simulink model "CRITIS_1_full"  (R2022b)
settings: Solver=VariableStepAuto  StartTime=0.0  StopTime=7  RelTol=1e-3
(part 10 of 13)

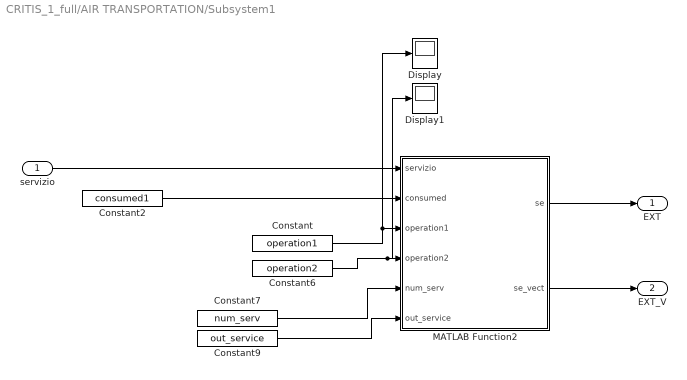
== system CRITIS_1_full/AIR TRANSPORTATION/Subsystem1 ==
  servizio : Inport
  Constant : Constant  Value=operation1
  Constant2 : Constant  Value=consumed1
  Constant6 : Constant  Value=operation2
  Constant7 : Constant  Value=num_serv
  Constant9 : Constant  Value=out_service
  Display : Display
  Display1 : Display
  MATLAB Function2 : MATLAB Function  TreatAsAtomicUnit=on
  EXT : Outport
  EXT_V : Outport  Port=2
  wires:
  Constant7/1 -> MATLAB Function2/5(num_serv)
  Constant9/1 -> MATLAB Function2/6(out_service)
  servizio/1 -> MATLAB Function2/1(servizio)
  Constant/1 -> Display/1, MATLAB Function2/3(operation1)
  Constant6/1 -> Display1/1, MATLAB Function2/4(operation2)
  MATLAB Function2/1(se) -> EXT/1
  MATLAB Function2/2(se_vect) -> EXT_V/1
  Constant2/1 -> MATLAB Function2/2(consumed)

== system CRITIS_1_full/AIR TRANSPORTATION/Subsystem10 ==
  servizio : Inport
  Constant : Constant  Value=operation1
  Constant2 : Constant  Value=consumed1
  Constant6 : Constant  Value=operation2
  Constant7 : Constant  Value=num_serv
  Constant9 : Constant  Value=out_service
  MATLAB Function2 : MATLAB Function  TreatAsAtomicUnit=on
  EXT : Outport
  EXT_V : Outport  Port=2
  wires:
  Constant7/1 -> MATLAB Function2/5(num_serv)
  Constant9/1 -> MATLAB Function2/6(out_service)
  servizio/1 -> MATLAB Function2/1(servizio)
  Constant/1 -> MATLAB Function2/3(operation1)
  Constant6/1 -> MATLAB Function2/4(operation2)
  MATLAB Function2/1(se) -> EXT/1
  MATLAB Function2/2(se_vect) -> EXT_V/1
  Constant2/1 -> MATLAB Function2/2(consumed)

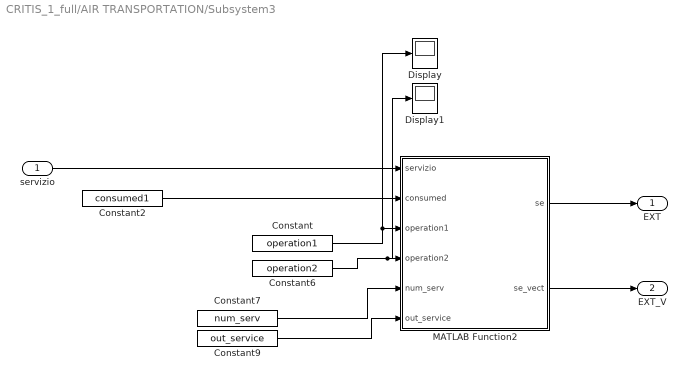
== system CRITIS_1_full/AIR TRANSPORTATION/Subsystem3 ==
  servizio : Inport
  Constant : Constant  Value=operation1
  Constant2 : Constant  Value=consumed1
  Constant6 : Constant  Value=operation2
  Constant7 : Constant  Value=num_serv
  Constant9 : Constant  Value=out_service
  Display : Display
  Display1 : Display
  MATLAB Function2 : MATLAB Function  TreatAsAtomicUnit=on
  EXT : Outport
  EXT_V : Outport  Port=2
  wires:
  Constant7/1 -> MATLAB Function2/5(num_serv)
  Constant9/1 -> MATLAB Function2/6(out_service)
  servizio/1 -> MATLAB Function2/1(servizio)
  Constant/1 -> Display/1, MATLAB Function2/3(operation1)
  Constant6/1 -> Display1/1, MATLAB Function2/4(operation2)
  MATLAB Function2/1(se) -> EXT/1
  MATLAB Function2/2(se_vect) -> EXT_V/1
  Constant2/1 -> MATLAB Function2/2(consumed)

== system CRITIS_1_full/AIR TRANSPORTATION/Subsystem4 ==
  servizio : Inport
  Constant : Constant  Value=operation1
  Constant2 : Constant  Value=consumed1
  Constant6 : Constant  Value=operation2
  Constant7 : Constant  Value=num_serv
  Constant9 : Constant  Value=out_service
  Display : Display
  Display1 : Display
  MATLAB Function2 : MATLAB Function  TreatAsAtomicUnit=on
  EXT : Outport
  EXT_V : Outport  Port=2
  wires:
  Constant7/1 -> MATLAB Function2/5(num_serv)
  Constant9/1 -> MATLAB Function2/6(out_service)
  servizio/1 -> MATLAB Function2/1(servizio)
  Constant/1 -> Display/1, MATLAB Function2/3(operation1)
  Constant6/1 -> Display1/1, MATLAB Function2/4(operation2)
  MATLAB Function2/1(se) -> EXT/1
  MATLAB Function2/2(se_vect) -> EXT_V/1
  Constant2/1 -> MATLAB Function2/2(consumed)

== system CRITIS_1_full/AIR TRANSPORTATION/Subsystem5 ==
  servizio : Inport
  Constant : Constant  Value=operation1
  Constant2 : Constant  Value=consumed1
  Constant6 : Constant  Value=operation2
  Constant7 : Constant  Value=num_serv
  Constant9 : Constant  Value=out_service
  Display : Display
  Display1 : Display
  MATLAB Function2 : MATLAB Function  TreatAsAtomicUnit=on
  EXT : Outport
  EXT_V : Outport  Port=2
  wires:
  Constant7/1 -> MATLAB Function2/5(num_serv)
  Constant9/1 -> MATLAB Function2/6(out_service)
  servizio/1 -> MATLAB Function2/1(servizio)
  Constant/1 -> Display/1, MATLAB Function2/3(operation1)
  Constant6/1 -> Display1/1, MATLAB Function2/4(operation2)
  MATLAB Function2/1(se) -> EXT/1
  MATLAB Function2/2(se_vect) -> EXT_V/1
  Constant2/1 -> MATLAB Function2/2(consumed)

== system CRITIS_1_full/AIR TRANSPORTATION/Subsystem6 ==
  servizio : Inport
  Constant : Constant  Value=operation1
  Constant2 : Constant  Value=consumed1
  Constant6 : Constant  Value=operation2
  Constant7 : Constant  Value=num_serv
  Constant9 : Constant  Value=out_service
  Display : Display
  Display1 : Display
  MATLAB Function2 : MATLAB Function  TreatAsAtomicUnit=on
  EXT : Outport
  EXT_V : Outport  Port=2
  wires:
  Constant7/1 -> MATLAB Function2/5(num_serv)
  Constant9/1 -> MATLAB Function2/6(out_service)
  servizio/1 -> MATLAB Function2/1(servizio)
  Constant/1 -> Display/1, MATLAB Function2/3(operation1)
  Constant6/1 -> Display1/1, MATLAB Function2/4(operation2)
  MATLAB Function2/1(se) -> EXT/1
  MATLAB Function2/2(se_vect) -> EXT_V/1
  Constant2/1 -> MATLAB Function2/2(consumed)

== system CRITIS_1_full/AIR TRANSPORTATION/Subsystem7 ==
  servizio : Inport
  Constant : Constant  Value=operation1
  Constant2 : Constant  Value=consumed1
  Constant6 : Constant  Value=operation2
  Constant7 : Constant  Value=num_serv
  Constant9 : Constant  Value=out_service
  Display : Display
  Display1 : Display
  MATLAB Function2 : MATLAB Function  TreatAsAtomicUnit=on
  EXT : Outport
  EXT_V : Outport  Port=2
  wires:
  Constant7/1 -> MATLAB Function2/5(num_serv)
  Constant9/1 -> MATLAB Function2/6(out_service)
  servizio/1 -> MATLAB Function2/1(servizio)
  Constant/1 -> Display/1, MATLAB Function2/3(operation1)
  Constant6/1 -> Display1/1, MATLAB Function2/4(operation2)
  MATLAB Function2/1(se) -> EXT/1
  MATLAB Function2/2(se_vect) -> EXT_V/1
  Constant2/1 -> MATLAB Function2/2(consumed)

== system CRITIS_1_full/AIR TRANSPORTATION/Subsystem8 ==
  servizio : Inport
  Constant : Constant  Value=operation1
  Constant2 : Constant  Value=consumed1
  Constant6 : Constant  Value=operation2
  Constant7 : Constant  Value=num_serv
  Constant9 : Constant  Value=out_service
  Display : Display
  Display1 : Display
  MATLAB Function2 : MATLAB Function  TreatAsAtomicUnit=on
  EXT : Outport
  EXT_V : Outport  Port=2
  wires:
  Constant7/1 -> MATLAB Function2/5(num_serv)
  Constant9/1 -> MATLAB Function2/6(out_service)
  servizio/1 -> MATLAB Function2/1(servizio)
  Constant/1 -> Display/1, MATLAB Function2/3(operation1)
  Constant6/1 -> Display1/1, MATLAB Function2/4(operation2)
  MATLAB Function2/1(se) -> EXT/1
  MATLAB Function2/2(se_vect) -> EXT_V/1
  Constant2/1 -> MATLAB Function2/2(consumed)

== system CRITIS_1_full/AIR TRANSPORTATION/Subsystem9 ==
  servizio : Inport
  Constant : Constant  Value=operation1
  Constant2 : Constant  Value=consumed1
  Constant6 : Constant  Value=operation2
  Constant7 : Constant  Value=num_serv
  Constant9 : Constant  Value=out_service
  MATLAB Function2 : MATLAB Function  TreatAsAtomicUnit=on
  EXT : Outport
  EXT_V : Outport  Port=2
  wires:
  Constant7/1 -> MATLAB Function2/5(num_serv)
  Constant9/1 -> MATLAB Function2/6(out_service)
  servizio/1 -> MATLAB Function2/1(servizio)
  Constant/1 -> MATLAB Function2/3(operation1)
  Constant6/1 -> MATLAB Function2/4(operation2)
  MATLAB Function2/1(se) -> EXT/1
  MATLAB Function2/2(se_vect) -> EXT_V/1
  Constant2/1 -> MATLAB Function2/2(consumed)

== system CRITIS_1_full/AIR TRANSPORTATION/delay ==
  in : Inport
  Clock : Clock
  Constant17 : Constant  Value=output
  Switch : Switch  Criteria=u2 > Threshold  Threshold=delay  SaturateOnIntegerOverflow=off  InputSameDT=off
  out : Outport
  wires:
  Switch/1 -> out/1
  Constant17/1 -> Switch/3
  in/1 -> Switch/1
  Clock/1 -> Switch/2

== system CRITIS_1_full/AIR TRANSPORTATION/delay1 ==
  in : Inport
  Clock : Clock
  Constant17 : Constant  Value=output
  Switch : Switch  Criteria=u2 > Threshold  Threshold=delay  SaturateOnIntegerOverflow=off  InputSameDT=off
  out : Outport
  wires:
  Switch/1 -> out/1
  Constant17/1 -> Switch/3
  in/1 -> Switch/1
  Clock/1 -> Switch/2

== system CRITIS_1_full/BANK 1/Subsystem1 ==
  servizio : Inport
  Constant : Constant  Value=operation1
  Constant2 : Constant  Value=consumed1
  Constant6 : Constant  Value=operation2
  Constant7 : Constant  Value=num_serv
  Constant9 : Constant  Value=out_service
  Display : Display
  Display1 : Display
  MATLAB Function2 : MATLAB Function  TreatAsAtomicUnit=on
  EXT : Outport
  EXT_V : Outport  Port=2
  wires:
  Constant7/1 -> MATLAB Function2/5(num_serv)
  Constant9/1 -> MATLAB Function2/6(out_service)
  servizio/1 -> MATLAB Function2/1(servizio)
  Constant/1 -> Display/1, MATLAB Function2/3(operation1)
  Constant6/1 -> Display1/1, MATLAB Function2/4(operation2)
  MATLAB Function2/1(se) -> EXT/1
  MATLAB Function2/2(se_vect) -> EXT_V/1
  Constant2/1 -> MATLAB Function2/2(consumed)

== system CRITIS_1_full/BANK 1/Subsystem2 ==
  servizio : Inport
  Constant : Constant  Value=operation1
  Constant2 : Constant  Value=consumed1
  Constant6 : Constant  Value=operation2
  Constant7 : Constant  Value=num_serv
  Constant9 : Constant  Value=out_service
  Display : Display
  Display1 : Display
  MATLAB Function2 : MATLAB Function  TreatAsAtomicUnit=on
  EXT : Outport
  EXT_V : Outport  Port=2
  wires:
  Constant7/1 -> MATLAB Function2/5(num_serv)
  Constant9/1 -> MATLAB Function2/6(out_service)
  servizio/1 -> MATLAB Function2/1(servizio)
  Constant/1 -> Display/1, MATLAB Function2/3(operation1)
  Constant6/1 -> Display1/1, MATLAB Function2/4(operation2)
  MATLAB Function2/1(se) -> EXT/1
  MATLAB Function2/2(se_vect) -> EXT_V/1
  Constant2/1 -> MATLAB Function2/2(consumed)

== system CRITIS_1_full/BANK 1/Subsystem3 ==
  servizio : Inport
  Constant : Constant  Value=operation1
  Constant2 : Constant  Value=consumed1
  Constant6 : Constant  Value=operation2
  Constant7 : Constant  Value=num_serv
  Constant9 : Constant  Value=out_service
  Display : Display
  Display1 : Display
  MATLAB Function2 : MATLAB Function  TreatAsAtomicUnit=on
  EXT : Outport
  EXT_V : Outport  Port=2
  wires:
  Constant7/1 -> MATLAB Function2/5(num_serv)
  Constant9/1 -> MATLAB Function2/6(out_service)
  servizio/1 -> MATLAB Function2/1(servizio)
  Constant/1 -> Display/1, MATLAB Function2/3(operation1)
  Constant6/1 -> Display1/1, MATLAB Function2/4(operation2)
  MATLAB Function2/1(se) -> EXT/1
  MATLAB Function2/2(se_vect) -> EXT_V/1
  Constant2/1 -> MATLAB Function2/2(consumed)

== system CRITIS_1_full/BANK 1/Subsystem4 ==
  servizio : Inport
  Constant : Constant  Value=operation1
  Constant2 : Constant  Value=consumed1
  Constant6 : Constant  Value=operation2
  Constant7 : Constant  Value=num_serv
  Constant9 : Constant  Value=out_service
  Display : Display
  Display1 : Display
  MATLAB Function2 : MATLAB Function  TreatAsAtomicUnit=on
  EXT : Outport
  EXT_V : Outport  Port=2
  wires:
  Constant7/1 -> MATLAB Function2/5(num_serv)
  Constant9/1 -> MATLAB Function2/6(out_service)
  servizio/1 -> MATLAB Function2/1(servizio)
  Constant/1 -> Display/1, MATLAB Function2/3(operation1)
  Constant6/1 -> Display1/1, MATLAB Function2/4(operation2)
  MATLAB Function2/1(se) -> EXT/1
  MATLAB Function2/2(se_vect) -> EXT_V/1
  Constant2/1 -> MATLAB Function2/2(consumed)

== system CRITIS_1_full/BANK 1/Subsystem5 ==
  servizio : Inport
  Constant : Constant  Value=operation1
  Constant2 : Constant  Value=consumed1
  Constant6 : Constant  Value=operation2
  Constant7 : Constant  Value=num_serv
  Constant9 : Constant  Value=out_service
  Display : Display
  Display1 : Display
  MATLAB Function2 : MATLAB Function  TreatAsAtomicUnit=on
  EXT : Outport
  EXT_V : Outport  Port=2
  wires:
  Constant7/1 -> MATLAB Function2/5(num_serv)
  Constant9/1 -> MATLAB Function2/6(out_service)
  servizio/1 -> MATLAB Function2/1(servizio)
  Constant/1 -> Display/1, MATLAB Function2/3(operation1)
  Constant6/1 -> Display1/1, MATLAB Function2/4(operation2)
  MATLAB Function2/1(se) -> EXT/1
  MATLAB Function2/2(se_vect) -> EXT_V/1
  Constant2/1 -> MATLAB Function2/2(consumed)

== system CRITIS_1_full/BANK 1/Subsystem6 ==
  servizio : Inport
  Constant : Constant  Value=operation1
  Constant2 : Constant  Value=consumed1
  Constant6 : Constant  Value=operation2
  Constant7 : Constant  Value=num_serv
  Constant9 : Constant  Value=out_service
  Display : Display
  Display1 : Display
  MATLAB Function2 : MATLAB Function  TreatAsAtomicUnit=on
  EXT : Outport
  EXT_V : Outport  Port=2
  wires:
  Constant7/1 -> MATLAB Function2/5(num_serv)
  Constant9/1 -> MATLAB Function2/6(out_service)
  servizio/1 -> MATLAB Function2/1(servizio)
  Constant/1 -> Display/1, MATLAB Function2/3(operation1)
  Constant6/1 -> Display1/1, MATLAB Function2/4(operation2)
  MATLAB Function2/1(se) -> EXT/1
  MATLAB Function2/2(se_vect) -> EXT_V/1
  Constant2/1 -> MATLAB Function2/2(consumed)

== system CRITIS_1_full/BANK 1/delay ==
  in : Inport
  Clock : Clock
  Constant17 : Constant  Value=output
  Switch : Switch  Criteria=u2 > Threshold  Threshold=delay  SaturateOnIntegerOverflow=off  InputSameDT=off
  out : Outport
  wires:
  Switch/1 -> out/1
  Constant17/1 -> Switch/3
  in/1 -> Switch/1
  Clock/1 -> Switch/2

== system CRITIS_1_full/BANK 1/delay1 ==
  in : Inport
  Clock : Clock
  Constant17 : Constant  Value=output
  Switch : Switch  Criteria=u2 > Threshold  Threshold=delay  SaturateOnIntegerOverflow=off  InputSameDT=off
  out : Outport
  wires:
  Switch/1 -> out/1
  Constant17/1 -> Switch/3
  in/1 -> Switch/1
  Clock/1 -> Switch/2

== system CRITIS_1_full/DEPARTMENT OF INDUSTRIAL DEVELOPMENT/Subsystem1 ==
  servizio : Inport
  Constant : Constant  Value=operation1
  Constant2 : Constant  Value=consumed1
  Constant6 : Constant  Value=operation2
  Constant7 : Constant  Value=num_serv
  Constant9 : Constant  Value=out_service
  Display : Display
  Display1 : Display
  MATLAB Function2 : MATLAB Function  TreatAsAtomicUnit=on
  EXT : Outport
  EXT_V : Outport  Port=2
  wires:
  Constant7/1 -> MATLAB Function2/5(num_serv)
  Constant9/1 -> MATLAB Function2/6(out_service)
  servizio/1 -> MATLAB Function2/1(servizio)
  Constant/1 -> Display/1, MATLAB Function2/3(operation1)
  Constant6/1 -> Display1/1, MATLAB Function2/4(operation2)
  MATLAB Function2/1(se) -> EXT/1
  MATLAB Function2/2(se_vect) -> EXT_V/1
  Constant2/1 -> MATLAB Function2/2(consumed)

== system CRITIS_1_full/DEPARTMENT OF INDUSTRIAL DEVELOPMENT/Subsystem2 ==
  servizio : Inport
  Constant : Constant  Value=operation1
  Constant2 : Constant  Value=consumed1
  Constant6 : Constant  Value=operation2
  Constant7 : Constant  Value=num_serv
  Constant9 : Constant  Value=out_service
  Display : Display
  Display1 : Display
  MATLAB Function2 : MATLAB Function  TreatAsAtomicUnit=on
  EXT : Outport
  EXT_V : Outport  Port=2
  wires:
  Constant7/1 -> MATLAB Function2/5(num_serv)
  Constant9/1 -> MATLAB Function2/6(out_service)
  servizio/1 -> MATLAB Function2/1(servizio)
  Constant/1 -> Display/1, MATLAB Function2/3(operation1)
  Constant6/1 -> Display1/1, MATLAB Function2/4(operation2)
  MATLAB Function2/1(se) -> EXT/1
  MATLAB Function2/2(se_vect) -> EXT_V/1
  Constant2/1 -> MATLAB Function2/2(consumed)

== system CRITIS_1_full/DEPARTMENT OF INDUSTRIAL DEVELOPMENT/Subsystem3 ==
  servizio : Inport
  Constant : Constant  Value=operation1
  Constant2 : Constant  Value=consumed1
  Constant6 : Constant  Value=operation2
  Constant7 : Constant  Value=num_serv
  Constant9 : Constant  Value=out_service
  Display : Display
  Display1 : Display
  MATLAB Function2 : MATLAB Function  TreatAsAtomicUnit=on
  EXT : Outport
  EXT_V : Outport  Port=2
  wires:
  Constant7/1 -> MATLAB Function2/5(num_serv)
  Constant9/1 -> MATLAB Function2/6(out_service)
  servizio/1 -> MATLAB Function2/1(servizio)
  Constant/1 -> Display/1, MATLAB Function2/3(operation1)
  Constant6/1 -> Display1/1, MATLAB Function2/4(operation2)
  MATLAB Function2/1(se) -> EXT/1
  MATLAB Function2/2(se_vect) -> EXT_V/1
  Constant2/1 -> MATLAB Function2/2(consumed)

== system CRITIS_1_full/DEPARTMENT OF INDUSTRIAL DEVELOPMENT/Subsystem4 ==
  servizio : Inport
  Constant : Constant  Value=operation1
  Constant2 : Constant  Value=consumed1
  Constant6 : Constant  Value=operation2
  Constant7 : Constant  Value=num_serv
  Constant9 : Constant  Value=out_service
  Display : Display
  Display1 : Display
  MATLAB Function2 : MATLAB Function  TreatAsAtomicUnit=on
  EXT : Outport
  EXT_V : Outport  Port=2
  wires:
  Constant7/1 -> MATLAB Function2/5(num_serv)
  Constant9/1 -> MATLAB Function2/6(out_service)
  servizio/1 -> MATLAB Function2/1(servizio)
  Constant/1 -> Display/1, MATLAB Function2/3(operation1)
  Constant6/1 -> Display1/1, MATLAB Function2/4(operation2)
  MATLAB Function2/1(se) -> EXT/1
  MATLAB Function2/2(se_vect) -> EXT_V/1
  Constant2/1 -> MATLAB Function2/2(consumed)

== system CRITIS_1_full/DEPARTMENT OF INDUSTRIAL DEVELOPMENT/Subsystem5 ==
  servizio : Inport
  Constant : Constant  Value=operation1
  Constant2 : Constant  Value=consumed1
  Constant6 : Constant  Value=operation2
  Constant7 : Constant  Value=num_serv
  Constant9 : Constant  Value=out_service
  Display : Display
  Display1 : Display
  MATLAB Function2 : MATLAB Function  TreatAsAtomicUnit=on
  EXT : Outport
  EXT_V : Outport  Port=2
  wires:
  Constant7/1 -> MATLAB Function2/5(num_serv)
  Constant9/1 -> MATLAB Function2/6(out_service)
  servizio/1 -> MATLAB Function2/1(servizio)
  Constant/1 -> Display/1, MATLAB Function2/3(operation1)
  Constant6/1 -> Display1/1, MATLAB Function2/4(operation2)
  MATLAB Function2/1(se) -> EXT/1
  MATLAB Function2/2(se_vect) -> EXT_V/1
  Constant2/1 -> MATLAB Function2/2(consumed)

== system CRITIS_1_full/DEPARTMENT OF INDUSTRIAL DEVELOPMENT/Subsystem6 ==
  servizio : Inport
  Constant : Constant  Value=operation1
  Constant2 : Constant  Value=consumed1
  Constant6 : Constant  Value=operation2
  Constant7 : Constant  Value=num_serv
  Constant9 : Constant  Value=out_service
  Display : Display
  Display1 : Display
  MATLAB Function2 : MATLAB Function  TreatAsAtomicUnit=on
  EXT : Outport
  EXT_V : Outport  Port=2
  wires:
  Constant7/1 -> MATLAB Function2/5(num_serv)
  Constant9/1 -> MATLAB Function2/6(out_service)
  servizio/1 -> MATLAB Function2/1(servizio)
  Constant/1 -> Display/1, MATLAB Function2/3(operation1)
  Constant6/1 -> Display1/1, MATLAB Function2/4(operation2)
  MATLAB Function2/1(se) -> EXT/1
  MATLAB Function2/2(se_vect) -> EXT_V/1
  Constant2/1 -> MATLAB Function2/2(consumed)

== system CRITIS_1_full/DEPARTMENT OF INDUSTRIAL DEVELOPMENT/delay ==
  in : Inport
  Clock : Clock
  Constant17 : Constant  Value=output
  Switch : Switch  Criteria=u2 > Threshold  Threshold=delay  SaturateOnIntegerOverflow=off  InputSameDT=off
  out : Outport
  wires:
  Switch/1 -> out/1
  Constant17/1 -> Switch/3
  in/1 -> Switch/1
  Clock/1 -> Switch/2

== system CRITIS_1_full/DEPARTMENT OF INDUSTRIAL DEVELOPMENT/delay1 ==
  in : Inport
  Clock : Clock
  Constant17 : Constant  Value=output
  Switch : Switch  Criteria=u2 > Threshold  Threshold=delay  SaturateOnIntegerOverflow=off  InputSameDT=off
  out : Outport
  wires:
  Switch/1 -> out/1
  Constant17/1 -> Switch/3
  in/1 -> Switch/1
  Clock/1 -> Switch/2

== system CRITIS_1_full/ENERGY PROVIDER 1/Subsystem1 ==
  servizio : Inport
  Constant : Constant  Value=operation1
  Constant2 : Constant  Value=consumed1
  Constant6 : Constant  Value=operation2
  Constant7 : Constant  Value=num_serv
  Constant9 : Constant  Value=out_service
  MATLAB Function2 : MATLAB Function  TreatAsAtomicUnit=on
  EXT : Outport
  EXT_V : Outport  Port=2
  wires:
  Constant7/1 -> MATLAB Function2/5(num_serv)
  Constant9/1 -> MATLAB Function2/6(out_service)
  servizio/1 -> MATLAB Function2/1(servizio)
  Constant/1 -> MATLAB Function2/3(operation1)
  Constant6/1 -> MATLAB Function2/4(operation2)
  MATLAB Function2/1(se) -> EXT/1
  MATLAB Function2/2(se_vect) -> EXT_V/1
  Constant2/1 -> MATLAB Function2/2(consumed)

== system CRITIS_1_full/ENERGY PROVIDER 1/Subsystem10 ==
  servizio : Inport
  Constant : Constant  Value=operation1
  Constant2 : Constant  Value=consumed1
  Constant6 : Constant  Value=operation2
  Constant7 : Constant  Value=num_serv
  Constant9 : Constant  Value=out_service
  MATLAB Function2 : MATLAB Function  TreatAsAtomicUnit=on
  EXT : Outport
  EXT_V : Outport  Port=2
  wires:
  Constant7/1 -> MATLAB Function2/5(num_serv)
  Constant9/1 -> MATLAB Function2/6(out_service)
  servizio/1 -> MATLAB Function2/1(servizio)
  Constant/1 -> MATLAB Function2/3(operation1)
  Constant6/1 -> MATLAB Function2/4(operation2)
  MATLAB Function2/1(se) -> EXT/1
  MATLAB Function2/2(se_vect) -> EXT_V/1
  Constant2/1 -> MATLAB Function2/2(consumed)

== system CRITIS_1_full/ENERGY PROVIDER 1/Subsystem2 ==
  servizio : Inport
  Constant : Constant  Value=operation1
  Constant2 : Constant  Value=consumed1
  Constant6 : Constant  Value=operation2
  Constant7 : Constant  Value=num_serv
  Constant9 : Constant  Value=out_service
  MATLAB Function2 : MATLAB Function  TreatAsAtomicUnit=on
  EXT : Outport
  EXT_V : Outport  Port=2
  wires:
  Constant7/1 -> MATLAB Function2/5(num_serv)
  Constant9/1 -> MATLAB Function2/6(out_service)
  servizio/1 -> MATLAB Function2/1(servizio)
  Constant/1 -> MATLAB Function2/3(operation1)
  Constant6/1 -> MATLAB Function2/4(operation2)
  MATLAB Function2/1(se) -> EXT/1
  MATLAB Function2/2(se_vect) -> EXT_V/1
  Constant2/1 -> MATLAB Function2/2(consumed)

== system CRITIS_1_full/ENERGY PROVIDER 1/Subsystem3 ==
  servizio : Inport
  Constant : Constant  Value=operation1
  Constant2 : Constant  Value=consumed1
  Constant6 : Constant  Value=operation2
  Constant7 : Constant  Value=num_serv
  Constant9 : Constant  Value=out_service
  Display : Display
  Display1 : Display
  MATLAB Function2 : MATLAB Function  TreatAsAtomicUnit=on
  EXT : Outport
  EXT_V : Outport  Port=2
  wires:
  Constant7/1 -> MATLAB Function2/5(num_serv)
  Constant9/1 -> MATLAB Function2/6(out_service)
  servizio/1 -> MATLAB Function2/1(servizio)
  Constant/1 -> Display/1, MATLAB Function2/3(operation1)
  Constant6/1 -> Display1/1, MATLAB Function2/4(operation2)
  MATLAB Function2/1(se) -> EXT/1
  MATLAB Function2/2(se_vect) -> EXT_V/1
  Constant2/1 -> MATLAB Function2/2(consumed)

== system CRITIS_1_full/ENERGY PROVIDER 1/Subsystem4 ==
  servizio : Inport
  Constant : Constant  Value=operation1
  Constant2 : Constant  Value=consumed1
  Constant6 : Constant  Value=operation2
  Constant7 : Constant  Value=num_serv
  Constant9 : Constant  Value=out_service
  MATLAB Function2 : MATLAB Function  TreatAsAtomicUnit=on
  EXT : Outport
  EXT_V : Outport  Port=2
  wires:
  Constant7/1 -> MATLAB Function2/5(num_serv)
  Constant9/1 -> MATLAB Function2/6(out_service)
  servizio/1 -> MATLAB Function2/1(servizio)
  Constant/1 -> MATLAB Function2/3(operation1)
  Constant6/1 -> MATLAB Function2/4(operation2)
  MATLAB Function2/1(se) -> EXT/1
  MATLAB Function2/2(se_vect) -> EXT_V/1
  Constant2/1 -> MATLAB Function2/2(consumed)

== system CRITIS_1_full/ENERGY PROVIDER 1/delay ==
  in : Inport
  Clock : Clock
  Constant17 : Constant  Value=output
  Switch : Switch  Criteria=u2 > Threshold  Threshold=delay  SaturateOnIntegerOverflow=off  InputSameDT=off
  out : Outport
  wires:
  Switch/1 -> out/1
  Constant17/1 -> Switch/3
  in/1 -> Switch/1
  Clock/1 -> Switch/2

== system CRITIS_1_full/ENERGY PROVIDER 1/delay1 ==
  in : Inport
  Clock : Clock
  Constant17 : Constant  Value=output
  Switch : Switch  Criteria=u2 > Threshold  Threshold=delay  SaturateOnIntegerOverflow=off  InputSameDT=off
  out : Outport
  wires:
  Switch/1 -> out/1
  Constant17/1 -> Switch/3
  in/1 -> Switch/1
  Clock/1 -> Switch/2

== system CRITIS_1_full/ENERGY PROVIDER 2/Subsystem1 ==
  servizio : Inport
  Constant : Constant  Value=operation1
  Constant2 : Constant  Value=consumed1
  Constant6 : Constant  Value=operation2
  Constant7 : Constant  Value=num_serv
  Constant9 : Constant  Value=out_service
  MATLAB Function2 : MATLAB Function  TreatAsAtomicUnit=on
  EXT : Outport
  EXT_V : Outport  Port=2
  wires:
  Constant7/1 -> MATLAB Function2/5(num_serv)
  Constant9/1 -> MATLAB Function2/6(out_service)
  servizio/1 -> MATLAB Function2/1(servizio)
  Constant/1 -> MATLAB Function2/3(operation1)
  Constant6/1 -> MATLAB Function2/4(operation2)
  MATLAB Function2/1(se) -> EXT/1
  MATLAB Function2/2(se_vect) -> EXT_V/1
  Constant2/1 -> MATLAB Function2/2(consumed)

== system CRITIS_1_full/ENERGY PROVIDER 2/Subsystem2 ==
  servizio : Inport
  Constant : Constant  Value=operation1
  Constant2 : Constant  Value=consumed1
  Constant6 : Constant  Value=operation2
  Constant7 : Constant  Value=num_serv
  Constant9 : Constant  Value=out_service
  MATLAB Function2 : MATLAB Function  TreatAsAtomicUnit=on
  EXT : Outport
  EXT_V : Outport  Port=2
  wires:
  Constant7/1 -> MATLAB Function2/5(num_serv)
  Constant9/1 -> MATLAB Function2/6(out_service)
  servizio/1 -> MATLAB Function2/1(servizio)
  Constant/1 -> MATLAB Function2/3(operation1)
  Constant6/1 -> MATLAB Function2/4(operation2)
  MATLAB Function2/1(se) -> EXT/1
  MATLAB Function2/2(se_vect) -> EXT_V/1
  Constant2/1 -> MATLAB Function2/2(consumed)

== system CRITIS_1_full/ENERGY PROVIDER 2/Subsystem4 ==
  servizio : Inport
  Constant : Constant  Value=operation1
  Constant2 : Constant  Value=consumed1
  Constant6 : Constant  Value=operation2
  Constant7 : Constant  Value=num_serv
  Constant9 : Constant  Value=out_service
  MATLAB Function2 : MATLAB Function  TreatAsAtomicUnit=on
  EXT : Outport
  EXT_V : Outport  Port=2
  wires:
  Constant7/1 -> MATLAB Function2/5(num_serv)
  Constant9/1 -> MATLAB Function2/6(out_service)
  servizio/1 -> MATLAB Function2/1(servizio)
  Constant/1 -> MATLAB Function2/3(operation1)
  Constant6/1 -> MATLAB Function2/4(operation2)
  MATLAB Function2/1(se) -> EXT/1
  MATLAB Function2/2(se_vect) -> EXT_V/1
  Constant2/1 -> MATLAB Function2/2(consumed)

== system CRITIS_1_full/ENERGY PROVIDER 2/Subsystem9 ==
  servizio : Inport
  Constant : Constant  Value=operation1
  Constant2 : Constant  Value=consumed1
  Constant6 : Constant  Value=operation2
  Constant7 : Constant  Value=num_serv
  Constant9 : Constant  Value=out_service
  MATLAB Function2 : MATLAB Function  TreatAsAtomicUnit=on
  EXT : Outport
  EXT_V : Outport  Port=2
  wires:
  Constant7/1 -> MATLAB Function2/5(num_serv)
  Constant9/1 -> MATLAB Function2/6(out_service)
  servizio/1 -> MATLAB Function2/1(servizio)
  Constant/1 -> MATLAB Function2/3(operation1)
  Constant6/1 -> MATLAB Function2/4(operation2)
  MATLAB Function2/1(se) -> EXT/1
  MATLAB Function2/2(se_vect) -> EXT_V/1
  Constant2/1 -> MATLAB Function2/2(consumed)

== system CRITIS_1_full/ENERGY PROVIDER 2/delay ==
  in : Inport
  Clock : Clock
  Constant17 : Constant  Value=output
  Switch : Switch  Criteria=u2 > Threshold  Threshold=delay  SaturateOnIntegerOverflow=off  InputSameDT=off
  out : Outport
  wires:
  Switch/1 -> out/1
  Constant17/1 -> Switch/3
  in/1 -> Switch/1
  Clock/1 -> Switch/2

== system CRITIS_1_full/ENERGY PROVIDER 2/delay1 ==
  in : Inport
  Clock : Clock
  Constant17 : Constant  Value=output
  Switch : Switch  Criteria=u2 > Threshold  Threshold=delay  SaturateOnIntegerOverflow=off  InputSameDT=off
  out : Outport
  wires:
  Switch/1 -> out/1
  Constant17/1 -> Switch/3
  in/1 -> Switch/1
  Clock/1 -> Switch/2

== system CRITIS_1_full/RAILWAYS/Subsystem1 ==
  servizio : Inport
  Constant : Constant  Value=operation1
  Constant2 : Constant  Value=consumed1
  Constant6 : Constant  Value=operation2
  Constant7 : Constant  Value=num_serv
  Constant9 : Constant  Value=out_service
  Display : Display
  Display1 : Display
  MATLAB Function2 : MATLAB Function  TreatAsAtomicUnit=on
  EXT : Outport
  EXT_V : Outport  Port=2
  wires:
  Constant7/1 -> MATLAB Function2/5(num_serv)
  Constant9/1 -> MATLAB Function2/6(out_service)
  servizio/1 -> MATLAB Function2/1(servizio)
  Constant/1 -> Display/1, MATLAB Function2/3(operation1)
  Constant6/1 -> Display1/1, MATLAB Function2/4(operation2)
  MATLAB Function2/1(se) -> EXT/1
  MATLAB Function2/2(se_vect) -> EXT_V/1
  Constant2/1 -> MATLAB Function2/2(consumed)

== system CRITIS_1_full/RAILWAYS/Subsystem10 ==
  servizio : Inport
  Constant : Constant  Value=operation1
  Constant2 : Constant  Value=consumed1
  Constant6 : Constant  Value=operation2
  Constant7 : Constant  Value=num_serv
  Constant9 : Constant  Value=out_service
  Display : Display
  Display1 : Display
  MATLAB Function2 : MATLAB Function  TreatAsAtomicUnit=on
  EXT : Outport
  EXT_V : Outport  Port=2
  wires:
  Constant7/1 -> MATLAB Function2/5(num_serv)
  Constant9/1 -> MATLAB Function2/6(out_service)
  servizio/1 -> MATLAB Function2/1(servizio)
  Constant/1 -> Display/1, MATLAB Function2/3(operation1)
  Constant6/1 -> Display1/1, MATLAB Function2/4(operation2)
  MATLAB Function2/1(se) -> EXT/1
  MATLAB Function2/2(se_vect) -> EXT_V/1
  Constant2/1 -> MATLAB Function2/2(consumed)

== system CRITIS_1_full/RAILWAYS/Subsystem11 ==
  servizio : Inport
  Constant : Constant  Value=operation1
  Constant2 : Constant  Value=consumed1
  Constant6 : Constant  Value=operation2
  Constant7 : Constant  Value=num_serv
  Constant9 : Constant  Value=out_service
  MATLAB Function2 : MATLAB Function  TreatAsAtomicUnit=on
  EXT : Outport
  EXT_V : Outport  Port=2
  wires:
  Constant7/1 -> MATLAB Function2/5(num_serv)
  Constant9/1 -> MATLAB Function2/6(out_service)
  servizio/1 -> MATLAB Function2/1(servizio)
  Constant/1 -> MATLAB Function2/3(operation1)
  Constant6/1 -> MATLAB Function2/4(operation2)
  MATLAB Function2/1(se) -> EXT/1
  MATLAB Function2/2(se_vect) -> EXT_V/1
  Constant2/1 -> MATLAB Function2/2(consumed)

== system CRITIS_1_full/RAILWAYS/Subsystem2 ==
  servizio : Inport
  Constant : Constant  Value=operation1
  Constant2 : Constant  Value=consumed1
  Constant6 : Constant  Value=operation2
  Constant7 : Constant  Value=num_serv
  Constant9 : Constant  Value=out_service
  Display : Display
  Display1 : Display
  MATLAB Function2 : MATLAB Function  TreatAsAtomicUnit=on
  EXT : Outport
  EXT_V : Outport  Port=2
  wires:
  Constant7/1 -> MATLAB Function2/5(num_serv)
  Constant9/1 -> MATLAB Function2/6(out_service)
  servizio/1 -> MATLAB Function2/1(servizio)
  Constant/1 -> Display/1, MATLAB Function2/3(operation1)
  Constant6/1 -> Display1/1, MATLAB Function2/4(operation2)
  MATLAB Function2/1(se) -> EXT/1
  MATLAB Function2/2(se_vect) -> EXT_V/1
  Constant2/1 -> MATLAB Function2/2(consumed)

== system CRITIS_1_full/RAILWAYS/Subsystem3 ==
  servizio : Inport
  Constant : Constant  Value=operation1
  Constant2 : Constant  Value=consumed1
  Constant6 : Constant  Value=operation2
  Constant7 : Constant  Value=num_serv
  Constant9 : Constant  Value=out_service
  Display : Display
  Display1 : Display
  MATLAB Function2 : MATLAB Function  TreatAsAtomicUnit=on
  EXT : Outport
  EXT_V : Outport  Port=2
  wires:
  Constant7/1 -> MATLAB Function2/5(num_serv)
  Constant9/1 -> MATLAB Function2/6(out_service)
  servizio/1 -> MATLAB Function2/1(servizio)
  Constant/1 -> Display/1, MATLAB Function2/3(operation1)
  Constant6/1 -> Display1/1, MATLAB Function2/4(operation2)
  MATLAB Function2/1(se) -> EXT/1
  MATLAB Function2/2(se_vect) -> EXT_V/1
  Constant2/1 -> MATLAB Function2/2(consumed)

== system CRITIS_1_full/RAILWAYS/Subsystem4 ==
  servizio : Inport
  Constant : Constant  Value=operation1
  Constant2 : Constant  Value=consumed1
  Constant6 : Constant  Value=operation2
  Constant7 : Constant  Value=num_serv
  Constant9 : Constant  Value=out_service
  Display : Display
  Display1 : Display
  MATLAB Function2 : MATLAB Function  TreatAsAtomicUnit=on
  EXT : Outport
  EXT_V : Outport  Port=2
  wires:
  Constant7/1 -> MATLAB Function2/5(num_serv)
  Constant9/1 -> MATLAB Function2/6(out_service)
  servizio/1 -> MATLAB Function2/1(servizio)
  Constant/1 -> Display/1, MATLAB Function2/3(operation1)
  Constant6/1 -> Display1/1, MATLAB Function2/4(operation2)
  MATLAB Function2/1(se) -> EXT/1
  MATLAB Function2/2(se_vect) -> EXT_V/1
  Constant2/1 -> MATLAB Function2/2(consumed)

== system CRITIS_1_full/RAILWAYS/Subsystem5 ==
  servizio : Inport
  Constant : Constant  Value=operation1
  Constant2 : Constant  Value=consumed1
  Constant6 : Constant  Value=operation2
  Constant7 : Constant  Value=num_serv
  Constant9 : Constant  Value=out_service
  Display : Display
  Display1 : Display
  MATLAB Function2 : MATLAB Function  TreatAsAtomicUnit=on
  EXT : Outport
  EXT_V : Outport  Port=2
  wires:
  Constant7/1 -> MATLAB Function2/5(num_serv)
  Constant9/1 -> MATLAB Function2/6(out_service)
  servizio/1 -> MATLAB Function2/1(servizio)
  Constant/1 -> Display/1, MATLAB Function2/3(operation1)
  Constant6/1 -> Display1/1, MATLAB Function2/4(operation2)
  MATLAB Function2/1(se) -> EXT/1
  MATLAB Function2/2(se_vect) -> EXT_V/1
  Constant2/1 -> MATLAB Function2/2(consumed)

== system CRITIS_1_full/RAILWAYS/Subsystem6 ==
  servizio : Inport
  Constant : Constant  Value=operation1
  Constant2 : Constant  Value=consumed1
  Constant6 : Constant  Value=operation2
  Constant7 : Constant  Value=num_serv
  Constant9 : Constant  Value=out_service
  Display : Display
  Display1 : Display
  MATLAB Function2 : MATLAB Function  TreatAsAtomicUnit=on
  EXT : Outport
  EXT_V : Outport  Port=2
  wires:
  Constant7/1 -> MATLAB Function2/5(num_serv)
  Constant9/1 -> MATLAB Function2/6(out_service)
  servizio/1 -> MATLAB Function2/1(servizio)
  Constant/1 -> Display/1, MATLAB Function2/3(operation1)
  Constant6/1 -> Display1/1, MATLAB Function2/4(operation2)
  MATLAB Function2/1(se) -> EXT/1
  MATLAB Function2/2(se_vect) -> EXT_V/1
  Constant2/1 -> MATLAB Function2/2(consumed)

== system CRITIS_1_full/RAILWAYS/Subsystem7 ==
  servizio : Inport
  Constant : Constant  Value=operation1
  Constant2 : Constant  Value=consumed1
  Constant6 : Constant  Value=operation2
  Constant7 : Constant  Value=num_serv
  Constant9 : Constant  Value=out_service
  Display : Display
  Display1 : Display
  MATLAB Function2 : MATLAB Function  TreatAsAtomicUnit=on
  EXT : Outport
  EXT_V : Outport  Port=2
  wires:
  Constant7/1 -> MATLAB Function2/5(num_serv)
  Constant9/1 -> MATLAB Function2/6(out_service)
  servizio/1 -> MATLAB Function2/1(servizio)
  Constant/1 -> Display/1, MATLAB Function2/3(operation1)
  Constant6/1 -> Display1/1, MATLAB Function2/4(operation2)
  MATLAB Function2/1(se) -> EXT/1
  MATLAB Function2/2(se_vect) -> EXT_V/1
  Constant2/1 -> MATLAB Function2/2(consumed)

== system CRITIS_1_full/RAILWAYS/Subsystem8 ==
  servizio : Inport
  Constant : Constant  Value=operation1
  Constant2 : Constant  Value=consumed1
  Constant6 : Constant  Value=operation2
  Constant7 : Constant  Value=num_serv
  Constant9 : Constant  Value=out_service
  Display : Display
  Display1 : Display
  MATLAB Function2 : MATLAB Function  TreatAsAtomicUnit=on
  EXT : Outport
  EXT_V : Outport  Port=2
  wires:
  Constant7/1 -> MATLAB Function2/5(num_serv)
  Constant9/1 -> MATLAB Function2/6(out_service)
  servizio/1 -> MATLAB Function2/1(servizio)
  Constant/1 -> Display/1, MATLAB Function2/3(operation1)
  Constant6/1 -> Display1/1, MATLAB Function2/4(operation2)
  MATLAB Function2/1(se) -> EXT/1
  MATLAB Function2/2(se_vect) -> EXT_V/1
  Constant2/1 -> MATLAB Function2/2(consumed)

== system CRITIS_1_full/RAILWAYS/Subsystem9 ==
  servizio : Inport
  Constant : Constant  Value=operation1
  Constant2 : Constant  Value=consumed1
  Constant6 : Constant  Value=operation2
  Constant7 : Constant  Value=num_serv
  Constant9 : Constant  Value=out_service
  Display : Display
  Display1 : Display
  MATLAB Function2 : MATLAB Function  TreatAsAtomicUnit=on
  EXT : Outport
  EXT_V : Outport  Port=2
  wires:
  Constant7/1 -> MATLAB Function2/5(num_serv)
  Constant9/1 -> MATLAB Function2/6(out_service)
  servizio/1 -> MATLAB Function2/1(servizio)
  Constant/1 -> Display/1, MATLAB Function2/3(operation1)
  Constant6/1 -> Display1/1, MATLAB Function2/4(operation2)
  MATLAB Function2/1(se) -> EXT/1
  MATLAB Function2/2(se_vect) -> EXT_V/1
  Constant2/1 -> MATLAB Function2/2(consumed)

== system CRITIS_1_full/RAILWAYS/delay ==
  in : Inport
  Clock : Clock
  Constant17 : Constant  Value=output
  Switch : Switch  Criteria=u2 > Threshold  Threshold=delay  SaturateOnIntegerOverflow=off  InputSameDT=off
  out : Outport
  wires:
  Switch/1 -> out/1
  Constant17/1 -> Switch/3
  in/1 -> Switch/1
  Clock/1 -> Switch/2

== system CRITIS_1_full/RAILWAYS/delay1 ==
  in : Inport
  Clock : Clock
  Constant17 : Constant  Value=output
  Switch : Switch  Criteria=u2 > Threshold  Threshold=delay  SaturateOnIntegerOverflow=off  InputSameDT=off
  out : Outport
  wires:
  Switch/1 -> out/1
  Constant17/1 -> Switch/3
  in/1 -> Switch/1
  Clock/1 -> Switch/2

== system CRITIS_1_full/TELCOMMUNICATIONS1/Subsystem1 ==
  servizio : Inport
  Constant : Constant  Value=operation1
  Constant2 : Constant  Value=consumed1
  Constant6 : Constant  Value=operation2
  Constant7 : Constant  Value=num_serv
  Constant9 : Constant  Value=out_service
  Display : Display
  Display1 : Display
  MATLAB Function2 : MATLAB Function  TreatAsAtomicUnit=on
  EXT : Outport
  EXT_V : Outport  Port=2
  wires:
  Constant7/1 -> MATLAB Function2/5(num_serv)
  Constant9/1 -> MATLAB Function2/6(out_service)
  servizio/1 -> MATLAB Function2/1(servizio)
  Constant/1 -> Display/1, MATLAB Function2/3(operation1)
  Constant6/1 -> Display1/1, MATLAB Function2/4(operation2)
  MATLAB Function2/1(se) -> EXT/1
  MATLAB Function2/2(se_vect) -> EXT_V/1
  Constant2/1 -> MATLAB Function2/2(consumed)

== system CRITIS_1_full/TELCOMMUNICATIONS1/Subsystem10 ==
  servizio : Inport
  Constant : Constant  Value=operation1
  Constant2 : Constant  Value=consumed1
  Constant6 : Constant  Value=operation2
  Constant7 : Constant  Value=num_serv
  Constant9 : Constant  Value=out_service
  MATLAB Function2 : MATLAB Function  TreatAsAtomicUnit=on
  EXT : Outport
  EXT_V : Outport  Port=2
  wires:
  Constant7/1 -> MATLAB Function2/5(num_serv)
  Constant9/1 -> MATLAB Function2/6(out_service)
  servizio/1 -> MATLAB Function2/1(servizio)
  Constant/1 -> MATLAB Function2/3(operation1)
  Constant6/1 -> MATLAB Function2/4(operation2)
  MATLAB Function2/1(se) -> EXT/1
  MATLAB Function2/2(se_vect) -> EXT_V/1
  Constant2/1 -> MATLAB Function2/2(consumed)

== system CRITIS_1_full/TELCOMMUNICATIONS1/Subsystem3 ==
  servizio : Inport
  Constant : Constant  Value=operation1
  Constant2 : Constant  Value=consumed1
  Constant6 : Constant  Value=operation2
  Constant7 : Constant  Value=num_serv
  Constant9 : Constant  Value=out_service
  Display : Display
  Display1 : Display
  MATLAB Function2 : MATLAB Function  TreatAsAtomicUnit=on
  EXT : Outport
  EXT_V : Outport  Port=2
  wires:
  Constant7/1 -> MATLAB Function2/5(num_serv)
  Constant9/1 -> MATLAB Function2/6(out_service)
  servizio/1 -> MATLAB Function2/1(servizio)
  Constant/1 -> Display/1, MATLAB Function2/3(operation1)
  Constant6/1 -> Display1/1, MATLAB Function2/4(operation2)
  MATLAB Function2/1(se) -> EXT/1
  MATLAB Function2/2(se_vect) -> EXT_V/1
  Constant2/1 -> MATLAB Function2/2(consumed)

== system CRITIS_1_full/TELCOMMUNICATIONS1/Subsystem5 ==
  servizio : Inport
  Constant : Constant  Value=operation1
  Constant2 : Constant  Value=consumed1
  Constant6 : Constant  Value=operation2
  Constant7 : Constant  Value=num_serv
  Constant9 : Constant  Value=out_service
  Display : Display
  Display1 : Display
  MATLAB Function2 : MATLAB Function  TreatAsAtomicUnit=on
  EXT : Outport
  EXT_V : Outport  Port=2
  wires:
  Constant7/1 -> MATLAB Function2/5(num_serv)
  Constant9/1 -> MATLAB Function2/6(out_service)
  servizio/1 -> MATLAB Function2/1(servizio)
  Constant/1 -> Display/1, MATLAB Function2/3(operation1)
  Constant6/1 -> Display1/1, MATLAB Function2/4(operation2)
  MATLAB Function2/1(se) -> EXT/1
  MATLAB Function2/2(se_vect) -> EXT_V/1
  Constant2/1 -> MATLAB Function2/2(consumed)

== system CRITIS_1_full/TELCOMMUNICATIONS1/Subsystem6 ==
  servizio : Inport
  Constant : Constant  Value=operation1
  Constant2 : Constant  Value=consumed1
  Constant6 : Constant  Value=operation2
  Constant7 : Constant  Value=num_serv
  Constant9 : Constant  Value=out_service
  MATLAB Function2 : MATLAB Function  TreatAsAtomicUnit=on
  EXT : Outport
  EXT_V : Outport  Port=2
  wires:
  Constant7/1 -> MATLAB Function2/5(num_serv)
  Constant9/1 -> MATLAB Function2/6(out_service)
  servizio/1 -> MATLAB Function2/1(servizio)
  Constant/1 -> MATLAB Function2/3(operation1)
  Constant6/1 -> MATLAB Function2/4(operation2)
  MATLAB Function2/1(se) -> EXT/1
  MATLAB Function2/2(se_vect) -> EXT_V/1
  Constant2/1 -> MATLAB Function2/2(consumed)
